simulink model "sampleModel233"  (R2021b)
settings: Solver=VariableStepAuto  StartTime=0.0  StopTime=10.0  RelTol=1e-3
undefined symbols (not defined in the file or in its folder): DiscIntNeverNeededParam
libraries: simulink x12, slpidlib x2
settings Model: Creator=user  LastModifiedBy=user

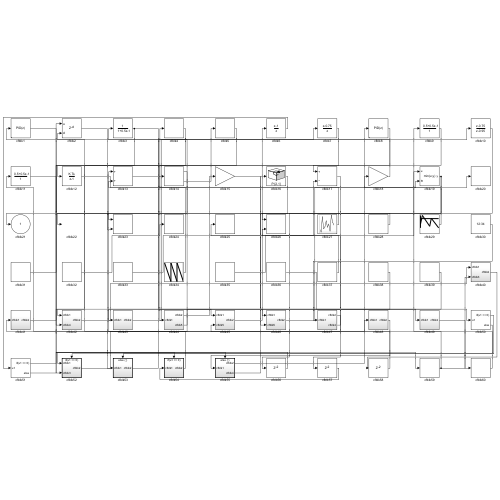
[thumbnail: Simulink's stored preview of the top-level diagram]
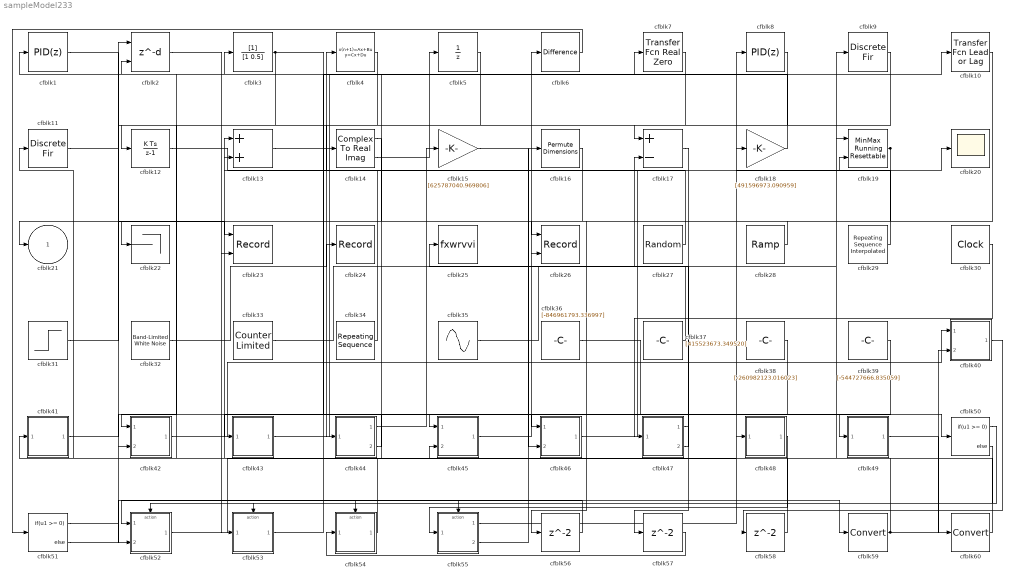
== system sampleModel233 ==
  cfblk1 : slpidlib/PID Controller  Controller=PID  Form=Parallel  TimeDomain=Discrete-time  UseExternalTs=off  SampleTime=1  IntegratorMethod=Forward Euler  FilterMethod=Forward Euler  ControllerParametersSource=internal  P=1  I=1  D=0  UseFilter=on  N=100  TunerSelectOption=Transfer Function Based (PID Tuner App)  InitialConditionSource=internal  InitialConditionForIntegrator=0  InitialConditionForFilter=0  DifferentiatorICPrevScaledInput=0  ExternalReset=none  TrackingMode=off  Kt=1  LimitOutput=off  SatLimitsSource=internal  UpperSaturationLimit=inf  LowerSaturationLimit=-inf  LinearizeAsGain=off  AntiWindupMode=none  Kb=1  POutMin=[]  POutMax=[]  IOutMin=[]  IOutMax=[]  DOutMin=[]  DOutMax=[]  NOutMin=[]  NOutMax=[]  SumOutMin=[]  SumOutMax=[]  SaturationOutMin=[]  SaturationOutMax=[]  PParamMin=[]  PParamMax=[]  IParamMin=[]  IParamMax=[]  DParamMin=[]  DParamMax=[]  NParamMin=[]  NParamMax=[]  KbParamMin=[]  KbParamMax=[]  KtParamMin=[]  KtParamMax=[]  KbOutMin=[]  KbOutMax=[]  KtOutMin=[]  KtOutMax=[]  IntegratorOutMin=[]  IntegratorOutMax=[]  FilterOutMin=[]  FilterOutMax=[]  SumI1OutMin=[]  SumI1OutMax=[]  SumI2OutMin=[]  SumI2OutMax=[]  SumI3OutMin=[]  SumI3OutMax=[]  SumI4OutMin=[]  SumI4OutMax=[]  SumDOutMin=[]  SumDOutMax=[]  DifferentiatorOutMin=[]  DifferentiatorOutMax=[]  FilterDiffOutCoefMin=[]  FilterDiffOutCoefMax=[]  ReciprocalOutMin=[]  ReciprocalOutMax=[]  SumDenOutMin=[]  SumDenOutMax=[]  SumNumOutMin=[]  SumNumOutMax=[]  DivideOutMin=[]  DivideOutMax=[]  UdiffTsProdOutMin=[]  UdiffTsProdOutMax=[]  NTsProdOutMin=[]  NTsProdOutMax=[]  UintegralTsProdOutMin=[]  UintegralTsProdOutMax=[]  UngainTsProdOutMin=[]  UngainTsProdOutMax=[]  IntegratorContinuousStateAttributes=''  IntegratorStateMustResolveToSignalObject=off  IntegratorRTWStateStorageClass=Auto  FilterContinuousStateAttributes=''  FilterStateMustResolveToSignalObject=off  FilterRTWStateStorageClass=Auto  ParallelPVariant=InternalParameters  IdealPVariant=Disabled  IVariant=InternalParameters  DVariant=InternalParameters  IntegratorVariant=Discrete  SatVariant=Disabled  AWVariant=Passthrough  PCopyVariant=Disabled  TRVariant=Disabled  FdbkBlocksVariant=Forward  IdealPFdbkVariant=Disabled  SatFdbkVariant=Disabled  DerivativeFilterVariant=ForwardEulerFilter  NVariant=InternalParameters  NCopyVariant=Disabled  FilterICVariant=InternalICsFilter  IntegratorICVariant=InternalICs  ExternalResetVariant=Disabled  TRSumVariant=Passthrough  SumFdbkVariant=Disabled  SumVariant=Sum_PID  TsampFilterVariant=InternalTs  TsampNgainVariant=Passthrough  TsampIntegralVariant=Passthrough  ExternalSaturationOutDataTypeStr=Inherit: Same as second input
  cfblk10 : simulink/Discrete/Transfer Fcn Lead or Lag  PoleZ=0.95  ZeroZ=0.75  ICPrevOutput=0.0  ICPrevInput=0.0  DoSatur=off
      settings: SourceProductBaseCode=SL
  cfblk11 : DiscreteFir  SampleTime=1
  cfblk12 : DiscreteIntegrator  ICPrevOutput=DiscIntNeverNeededParam  ICPrevScaledInput=DiscIntNeverNeededParam
  cfblk13 : Sum
  cfblk14 : ComplexToRealImag
  cfblk15 : Gain  Gain=[625787040.969806]
  cfblk16 : PermuteDimensions
  cfblk17 : Sum  Inputs=+-
  cfblk18 : Gain  Gain=[491596973.090959]
  cfblk19 : simulink/Math Operations/MinMax Running Resettable  Function=min  vinit=0.0
  cfblk2 : Delay  DelayLengthSource=Input port  SampleTime=1
      settings: InputPortMap=u0,p1
  cfblk20 : Scope
  cfblk22 : Terminator
  cfblk23 : Record  FileSettingsInternal="{\"entries\":[{\"content\":{\"excelSettings\":{\"content\":{},\"type\":\"Streamout.ExcelSettings\"}},\"type\":\"Streamout.FileSettingStorage\",\"uuid\":\"e433c555-253d-4f97-8293-8df6897d1aa0\"}],\"packageUris\":[\"http://schema.mathworks.com/mf0/streamout_blocks/R2020a\"],\"version\":\"1.0\"}"  Layout=[1 1]  SignalsInternal="{\"entries\":[{\"content\":{\"signals\":[{\"content\":{\"blockPath\":[\"sampleModel233/cfblk23\"],\"channel\":[],\"dimensions\":[1],\"domain\":\"sampleModel233/cfblk23\",\"lineColor\":\"#a2142f\",\"plots\":[1],\"port\":1,\"sid\":[\"\"],\"signalID\":9202,\"signalName\":\"cfblk1\"},\"type\":\"RecordBlkView.Signal\",\"uuid\":\"cc64b0a1-a71a-4532-a88e-b589344ca991\"},{\"content\":{\"blockPath\":[\"sampleModel233/cfblk23\"],\"channel\":[],\"dimensions\":[1],\"domain\":\"sampleModel233/cfblk23\",\"lineColor\":\"#139fff\",\"plots\":[1],\"port\":2,\"sid\":[\"\"],\"signalID\":9206,\"signalName\":\"cfblk10\"},\"type\":\"RecordBlkView.Signal\",\"uuid\":\"da4b2b64-4f55-4950-85e9-c9e6e136151f\"}]},\"type\":\"RecordBlkView.InputSignals\",\"uuid\":\"892f67e6-a918-4179-bd59-0d048ec73e92\"}],\"packageUris\":[\"http://schema.mathworks.com/mf0/streamout_blocks/R2020a\"],\"version\":\"1.0\"}"  VisualizationBindings="{\"xyplotplugin\":{\"info\":[{\"series\":[{\"bindingParametersList\":[{\"parameter\":\"X-Axis\",\"signalID\":9202,\"signalName\":\"cfblk1\"},{\"parameter\":\"Y-Axis\",\"signalID\":9206,\"signalName\":\"cfblk10\"}],\"seriesID\":50401}],\"subplotID\":1}]}}"  CompatibilityTag=XY
  cfblk24 : Record  FileSettingsInternal="{\"entries\":[{\"content\":{\"excelSettings\":{\"content\":{},\"type\":\"Streamout.ExcelSettings\"}},\"type\":\"Streamout.FileSettingStorage\",\"uuid\":\"70fc0ae0-eaa1-45bd-bad8-642bd3898e6d\"}],\"packageUris\":[\"http://schema.mathworks.com/mf0/streamout_blocks/R2020a\"],\"version\":\"1.0\"}"  SignalsInternal="{\"entries\":[{\"content\":{\"signals\":[{\"content\":{\"blockPath\":[\"sampleModel233/cfblk24\"],\"channel\":[],\"dimensions\":[1],\"domain\":\"sampleModel233/cfblk24\",\"lineColor\":\"#139fff\",\"plots\":[1],\"port\":1,\"sid\":[\"\"],\"signalID\":9210,\"signalName\":\"cfblk32\"},\"type\":\"RecordBlkView.Signal\",\"uuid\":\"13c7f2aa-63d0-4c70-a1a7-97bc0ddb1392\"}]},\"type\":\"RecordBlkView.InputSignals\",\"uuid\":\"2fd97512-d4e6-46da-8c1d-3fc5dd045031\"}],\"packageUris\":[\"http://schema.mathworks.com/mf0/streamout_blocks/R2020a\"],\"version\":\"1.0\"}"  VisualizationBindings="{\"sparklinesplugin\":{\"info\":[{\"bindingParametersList\":[],\"subplotID\":1}]}}"
  cfblk25 : ToWorkspace  VariableName=fxwrvvi  SaveFormat=Timeseries  SampleTime=-1
  cfblk26 : Record  FileSettingsInternal="{\"entries\":[{\"content\":{\"excelSettings\":{\"content\":{},\"type\":\"Streamout.ExcelSettings\"}},\"type\":\"Streamout.FileSettingStorage\",\"uuid\":\"40fa8434-3017-4f19-81d4-f6b42852243f\"}],\"packageUris\":[\"http://schema.mathworks.com/mf0/streamout_blocks/R2020a\"],\"version\":\"1.0\"}"  Layout=[1 1]  SignalsInternal="{\"entries\":[{\"content\":{\"signals\":[{\"content\":{\"blockPath\":[\"sampleModel233/cfblk26\"],\"channel\":[],\"dimensions\":[1],\"domain\":\"sampleModel233/cfblk26\",\"lineColor\":\"#a2142f\",\"plots\":[1],\"port\":1,\"sid\":[\"\"],\"signalID\":9194,\"signalName\":\"cfblk28\"},\"type\":\"RecordBlkView.Signal\",\"uuid\":\"12f54125-0b3f-4167-9e98-b6753dddff8c\"},{\"content\":{\"blockPath\":[\"sampleModel233/cfblk26\"],\"channel\":[],\"dimensions\":[1],\"domain\":\"sampleModel233/cfblk26\",\"lineColor\":\"#139fff\",\"plots\":[1],\"port\":2,\"sid\":[\"\"],\"signalID\":9198,\"signalName\":\"cfblk47:2\"},\"type\":\"RecordBlkView.Signal\",\"uuid\":\"8ebd628b-74f3-4bb5-a465-ecb9d8ba75bf\"}]},\"type\":\"RecordBlkView.InputSignals\",\"uuid\":\"582ba211-169a-45ed-b58f-cc2af242cb11\"}],\"packageUris\":[\"http://schema.mathworks.com/mf0/streamout_blocks/R2020a\"],\"version\":\"1.0\"}"  VisualizationBindings="{\"xyplotplugin\":{\"info\":[{\"series\":[{\"bindingParametersList\":[{\"parameter\":\"X-Axis\",\"signalID\":9194,\"signalName\":\"cfblk28\"},{\"parameter\":\"Y-Axis\",\"signalID\":9198,\"signalName\":\"cfblk47:2\"}],\"seriesID\":20120}],\"subplotID\":1}]}}"  CompatibilityTag=XY
  cfblk27 : UniformRandomNumber  Minimum=[-4695507842.631408]  Maximum=[7164626324.547557]  Seed=[49075245.000000]  SampleTime=0.1
  cfblk28 : simulink/Sources/Ramp  slope=[-6346.107592]  start=[25.028759]  InitialOutput=[197981.904005]
  cfblk29 : simulink/Sources/Repeating Sequence Interpolated  OutValues=[-604105355.408719, 351627457.946515, -825257484.971985, 24988787.029643, -988722990.351069]  TimeValues=[0 0.1 0.5 0.6 1].'  LookUpMeth=Use Input Below  tsamp=0.01  OutMin=[]  OutMax=[]  OutDataTypeStr=double  OutputDataTypeScalingMode=double  OutDataType=fixdt(0,8)  OutScaling=2^-10
  cfblk3 : DiscreteFilter  SampleTime=1
  cfblk30 : DigitalClock
  cfblk31 : Step  Time=[5.000000]  Before=[-923331049.645190]  After=[146956045.634263]  SampleTime=0
  cfblk32 : simulink/Sources/Band-Limited White Noise  Cov=[272015035.903703]  Ts=0.1  seed=[5658208015.000000]
  cfblk33 : simulink/Sources/Counter Limited  uplimit=[322.000000]  tsamp=-1
  cfblk34 : simulink/Sources/Repeating Sequence  rep_seq_t=[0 2]  rep_seq_y=[143914466.926018, -976614914.177584]
  cfblk35 : Sin  Amplitude=[-571808846.141234]  Bias=[-474539122.793349]  SampleTime=0
  cfblk36 : Constant  Value=[-846961793.336997]  SampleTime=1
  cfblk37 : Constant  Value=[415523673.349520]  SampleTime=1
  cfblk38 : Constant  Value=[-260982123.016023]  SampleTime=1
  cfblk39 : Constant  Value=[-544727666.835059]  SampleTime=1
  cfblk4 : DiscreteStateSpace
  cfblk40 : Subsystem
  cfblk41 : Subsystem
  cfblk42 : Subsystem
  cfblk43 : Subsystem
  cfblk44 : Subsystem
  cfblk45 : Subsystem
  cfblk46 : Subsystem
  cfblk47 : Subsystem
  cfblk48 : Subsystem
  cfblk49 : Subsystem
  cfblk5 : UnitDelay  HasFrameUpgradeWarning=on
  cfblk50 : If  IfExpression=u1 >= 0  SampleTime=1
  cfblk51 : If  IfExpression=u1 >= 0  SampleTime=1
  cfblk52 : Subsystem  TreatAsAtomicUnit=on
  cfblk53 : Subsystem  TreatAsAtomicUnit=on
  cfblk54 : Subsystem  TreatAsAtomicUnit=on
  cfblk55 : Subsystem  TreatAsAtomicUnit=on
  cfblk56 : Delay  SampleTime=1
  cfblk57 : Delay  SampleTime=1
  cfblk58 : Delay  SampleTime=1
  cfblk59 : DataTypeConversion
  cfblk6 : simulink/Discrete/Difference  ICPrevInput=0.0  OutMin=[]  OutMax=[]  OutDataTypeStr=Inherit: Inherit via back propagation  OutDataType=fixdt(1, 16)  OutScaling=2^-10  DoSatur=off
  cfblk60 : DataTypeConversion
  cfblk7 : simulink/Discrete/Transfer Fcn Real Zero  ZeroZ=0.75  ICPrevInput=0.0  DoSatur=off
      settings: SourceProductBaseCode=SL
  cfblk8 : slpidlib/PID Controller  Controller=PID  Form=Parallel  TimeDomain=Discrete-time  UseExternalTs=off  SampleTime=1  IntegratorMethod=Forward Euler  FilterMethod=Forward Euler  ControllerParametersSource=internal  P=1  I=1  D=0  UseFilter=on  N=100  TunerSelectOption=Transfer Function Based (PID Tuner App)  InitialConditionSource=internal  InitialConditionForIntegrator=0  InitialConditionForFilter=0  DifferentiatorICPrevScaledInput=0  ExternalReset=none  TrackingMode=off  Kt=1  LimitOutput=off  SatLimitsSource=internal  UpperSaturationLimit=inf  LowerSaturationLimit=-inf  LinearizeAsGain=off  AntiWindupMode=none  Kb=1  POutMin=[]  POutMax=[]  IOutMin=[]  IOutMax=[]  DOutMin=[]  DOutMax=[]  NOutMin=[]  NOutMax=[]  SumOutMin=[]  SumOutMax=[]  SaturationOutMin=[]  SaturationOutMax=[]  PParamMin=[]  PParamMax=[]  IParamMin=[]  IParamMax=[]  DParamMin=[]  DParamMax=[]  NParamMin=[]  NParamMax=[]  KbParamMin=[]  KbParamMax=[]  KtParamMin=[]  KtParamMax=[]  KbOutMin=[]  KbOutMax=[]  KtOutMin=[]  KtOutMax=[]  IntegratorOutMin=[]  IntegratorOutMax=[]  FilterOutMin=[]  FilterOutMax=[]  SumI1OutMin=[]  SumI1OutMax=[]  SumI2OutMin=[]  SumI2OutMax=[]  SumI3OutMin=[]  SumI3OutMax=[]  SumI4OutMin=[]  SumI4OutMax=[]  SumDOutMin=[]  SumDOutMax=[]  DifferentiatorOutMin=[]  DifferentiatorOutMax=[]  FilterDiffOutCoefMin=[]  FilterDiffOutCoefMax=[]  ReciprocalOutMin=[]  ReciprocalOutMax=[]  SumDenOutMin=[]  SumDenOutMax=[]  SumNumOutMin=[]  SumNumOutMax=[]  DivideOutMin=[]  DivideOutMax=[]  UdiffTsProdOutMin=[]  UdiffTsProdOutMax=[]  NTsProdOutMin=[]  NTsProdOutMax=[]  UintegralTsProdOutMin=[]  UintegralTsProdOutMax=[]  UngainTsProdOutMin=[]  UngainTsProdOutMax=[]  IntegratorContinuousStateAttributes=''  IntegratorStateMustResolveToSignalObject=off  IntegratorRTWStateStorageClass=Auto  FilterContinuousStateAttributes=''  FilterStateMustResolveToSignalObject=off  FilterRTWStateStorageClass=Auto  ParallelPVariant=InternalParameters  IdealPVariant=Disabled  IVariant=InternalParameters  DVariant=InternalParameters  IntegratorVariant=Discrete  SatVariant=Disabled  AWVariant=Passthrough  PCopyVariant=Disabled  TRVariant=Disabled  FdbkBlocksVariant=Forward  IdealPFdbkVariant=Disabled  SatFdbkVariant=Disabled  DerivativeFilterVariant=ForwardEulerFilter  NVariant=InternalParameters  NCopyVariant=Disabled  FilterICVariant=InternalICsFilter  IntegratorICVariant=InternalICs  ExternalResetVariant=Disabled  TRSumVariant=Passthrough  SumFdbkVariant=Disabled  SumVariant=Sum_PID  TsampFilterVariant=InternalTs  TsampNgainVariant=Passthrough  TsampIntegralVariant=Passthrough  ExternalSaturationOutDataTypeStr=Inherit: Same as second input
  cfblk9 : DiscreteFir  SampleTime=1
  cfblk21 : Outport
  wires:
  cfblk43/1(cfblk2) -> cfblk10/1
  cfblk39/1 -> cfblk41/1(cfblk1)
  cfblk37/1 -> cfblk25/1
  cfblk42/1(cfblk2) -> cfblk40/1(cfblk1)
  cfblk11/1 -> cfblk59/1
  cfblk55/1(cfblk2) -> cfblk8/1
  cfblk14/1 -> cfblk22/1
  cfblk3/1 -> cfblk42/1(cfblk1), cfblk46/1(cfblk1)
  cfblk19/1 -> cfblk46/2(cfblk5), cfblk56/1
  cfblk8/1 -> cfblk17/1
  cfblk6/1 -> cfblk51/1
  cfblk16/1 -> cfblk21/1
  cfblk45/1(cfblk2) -> cfblk6/1
  cfblk46/1(cfblk2) -> cfblk20/1
  cfblk7/1 -> cfblk44/1(cfblk1)
  cfblk30/1 -> cfblk47/1(cfblk1)
  cfblk28/1 -> cfblk26/1
  cfblk32/1 -> cfblk24/1
  cfblk4/1 -> cfblk42/2(cfblk4)
  cfblk5/1 -> cfblk12/1
  cfblk12/1 -> cfblk19/2
  cfblk36/1 -> cfblk50/1
  cfblk52/1(cfblk2) -> cfblk48/1(cfblk1)
  cfblk41/1(cfblk2) -> cfblk45/1(cfblk1)
  cfblk55/2(cfblk4) -> cfblk16/1
  cfblk54/1(cfblk2) -> cfblk13/1
  cfblk33/1 -> cfblk17/2
  cfblk13/1 -> cfblk4/1
  cfblk14/2 -> cfblk5/1
  cfblk34/1 -> cfblk14/1
  cfblk15/1 -> cfblk49/1(cfblk1)
  cfblk44/1(cfblk2) -> cfblk15/1
  cfblk2/1 -> cfblk53/1(cfblk1)
  cfblk31/1 -> cfblk2/1
  cfblk29/1 -> cfblk18/1
  cfblk18/1 -> cfblk1/1
  cfblk47/1(cfblk2) -> cfblk45/2(cfblk5)
  cfblk1/1 -> cfblk23/1
  cfblk27/1 -> cfblk13/2
  cfblk10/1 -> cfblk23/2
  cfblk35/1 -> cfblk9/1
  cfblk48/1(cfblk2) -> cfblk55/1(cfblk1)
  cfblk53/1(cfblk2) -> cfblk7/1
  cfblk9/1 -> cfblk52/2(cfblk3)
  cfblk44/2(cfblk5) -> cfblk3/1
  cfblk47/2(cfblk4) -> cfblk26/2
  cfblk38/1 -> cfblk43/1(cfblk1)
  cfblk50/1 -> cfblk52/Action
  cfblk50/2 -> cfblk53/Action
  cfblk51/1 -> cfblk54/Action
  cfblk51/2 -> cfblk55/Action
  cfblk56/1 -> cfblk52/1(cfblk1)
  cfblk17/1 -> cfblk57/1
  cfblk57/1 -> cfblk54/1(cfblk1)
  cfblk40/1(cfblk2) -> cfblk58/1
  cfblk58/1 -> cfblk2/2
  cfblk59/1 -> cfblk40/2(cfblk3), cfblk19/1
  cfblk49/1(cfblk2) -> cfblk60/1
  cfblk60/1 -> cfblk11/1

== system sampleModel233/cfblk40 ==
  cfblk1 : Inport
  cfblk3 : Inport  Port=2
  cfblk2 : Outport
  wires:
  cfblk3/1 -> cfblk2/1

== system sampleModel233/cfblk41 ==
  cfblk1 : Inport
  cfblk3 : Gain  Gain=[-52154582.022978]
  cfblk2 : Outport
  wires:
  cfblk1/1 -> cfblk2/1, cfblk3/1

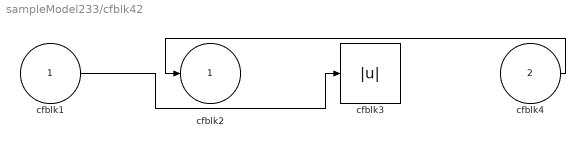
== system sampleModel233/cfblk42 ==
  cfblk1 : Inport
  cfblk4 : Inport  Port=2
  cfblk3 : Abs
  cfblk2 : Outport
  wires:
  cfblk4/1 -> cfblk2/1
  cfblk1/1 -> cfblk3/1

== system sampleModel233/cfblk43 ==
  cfblk1 : Inport
  cfblk3 : Gain  Gain=[-497471143.273681]
  cfblk2 : Outport
  wires:
  cfblk3/1 -> cfblk2/1
  cfblk1/1 -> cfblk3/1

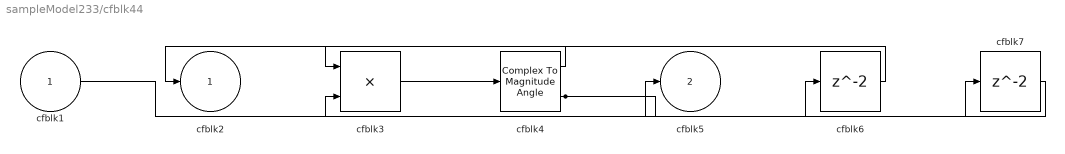
== system sampleModel233/cfblk44 ==
  cfblk1 : Inport
  cfblk3 : Product  Inputs=**
  cfblk4 : ComplexToMagnitudeAngle
  cfblk6 : Delay  SampleTime=1
  cfblk7 : Delay  SampleTime=1
  cfblk2 : Outport
  cfblk5 : Outport  Port=2
  wires:
  cfblk4/1 -> cfblk2/1
  cfblk3/1 -> cfblk4/1
  cfblk1/1 -> cfblk5/1
  cfblk4/2 -> cfblk6/1, cfblk7/1
  cfblk6/1 -> cfblk3/1
  cfblk7/1 -> cfblk3/2

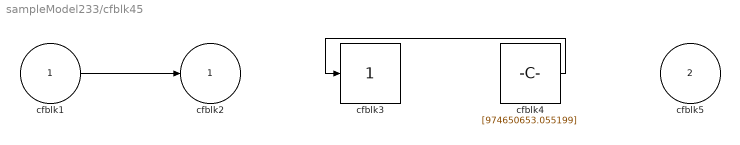
== system sampleModel233/cfblk45 ==
  cfblk1 : Inport
  cfblk5 : Inport  Port=2
  cfblk3 : simulink/Math Operations/Slider Gain  gain=1  low=0  high=2
  cfblk4 : Constant  Value=[974650653.055199]  SampleTime=1
  cfblk2 : Outport
  wires:
  cfblk4/1 -> cfblk3/1
  cfblk1/1 -> cfblk2/1

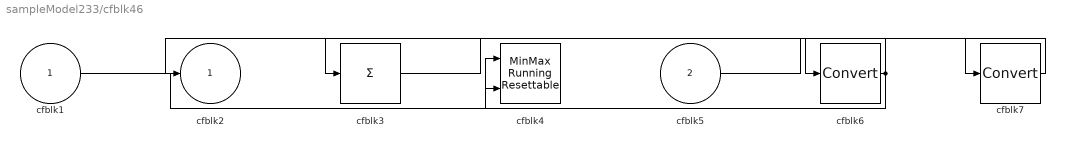
== system sampleModel233/cfblk46 ==
  cfblk1 : Inport
  cfblk5 : Inport  Port=2
  cfblk3 : Sum  Inputs=+
  cfblk4 : simulink/Math Operations/MinMax Running Resettable  Function=min  vinit=0.0
  cfblk6 : DataTypeConversion
  cfblk7 : DataTypeConversion
  cfblk2 : Outport
  wires:
  cfblk1/1 -> cfblk4/1
  cfblk3/1 -> cfblk6/1
  cfblk6/1 -> cfblk4/2, cfblk2/1
  cfblk5/1 -> cfblk7/1
  cfblk7/1 -> cfblk3/1

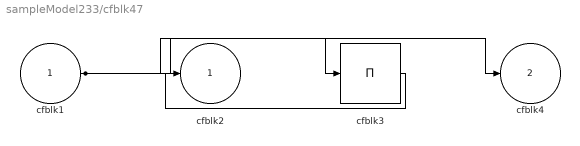
== system sampleModel233/cfblk47 ==
  cfblk1 : Inport
  cfblk3 : Product  Inputs=*
  cfblk2 : Outport
  cfblk4 : Outport  Port=2
  wires:
  cfblk1/1 -> cfblk3/1, cfblk4/1
  cfblk3/1 -> cfblk2/1

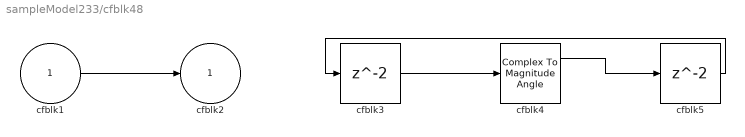
== system sampleModel233/cfblk48 ==
  cfblk1 : Inport
  cfblk3 : Delay  SampleTime=1
  cfblk4 : ComplexToMagnitudeAngle
  cfblk5 : Delay  SampleTime=1
  cfblk2 : Outport
  wires:
  cfblk3/1 -> cfblk4/1
  cfblk1/1 -> cfblk2/1
  cfblk4/1 -> cfblk5/1
  cfblk5/1 -> cfblk3/1

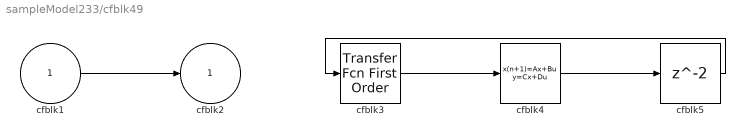
== system sampleModel233/cfblk49 ==
  cfblk1 : Inport
  cfblk3 : simulink/Discrete/Transfer Fcn First Order  PoleZ=0.95  ICPrevOutput=0.0  DoSatur=off
  cfblk4 : DiscreteStateSpace
  cfblk5 : Delay  SampleTime=1
  cfblk2 : Outport
  wires:
  cfblk3/1 -> cfblk4/1
  cfblk1/1 -> cfblk2/1
  cfblk4/1 -> cfblk5/1
  cfblk5/1 -> cfblk3/1

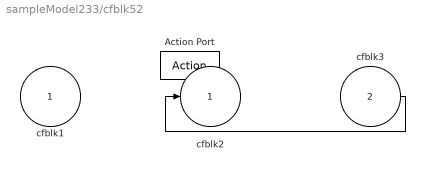
== system sampleModel233/cfblk52 ==
  cfblk1 : Inport
  cfblk3 : Inport  Port=2
  Action Port : ActionPort  ActionPortLabel=if(u1 >= 0)
  cfblk2 : Outport
  wires:
  cfblk3/1 -> cfblk2/1

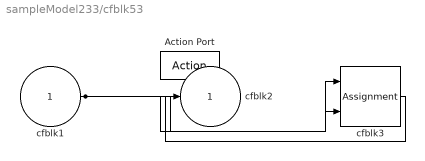
== system sampleModel233/cfblk53 ==
  cfblk1 : Inport
  Action Port : ActionPort  ActionPortLabel=else
  cfblk3 : Assignment  DiagnosticForDimensions=Warning  IndexOptions=Index vector (dialog)  Indices=1  OutputSizes=1
  cfblk2 : Outport
  wires:
  cfblk1/1 -> cfblk3/1, cfblk3/2
  cfblk3/1 -> cfblk2/1

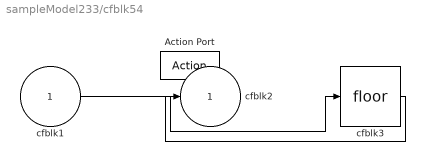
== system sampleModel233/cfblk54 ==
  cfblk1 : Inport
  Action Port : ActionPort  ActionPortLabel=if(u1 >= 0)
  cfblk3 : Rounding
  cfblk2 : Outport
  wires:
  cfblk1/1 -> cfblk3/1
  cfblk3/1 -> cfblk2/1

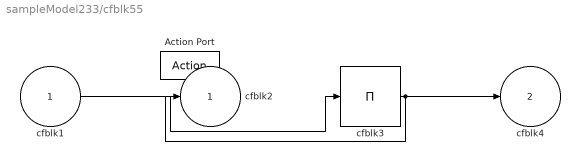
== system sampleModel233/cfblk55 ==
  cfblk1 : Inport
  Action Port : ActionPort  ActionPortLabel=else
  cfblk3 : Product  Inputs=*
  cfblk2 : Outport
  cfblk4 : Outport  Port=2
  wires:
  cfblk1/1 -> cfblk3/1
  cfblk3/1 -> cfblk2/1, cfblk4/1
